simulink model "ball_trajectory"  (R2026a)
settings: Solver=VariableStepAuto  StopTime=5
settings Model: Creator=tdxt  LastModifiedBy=tdxt

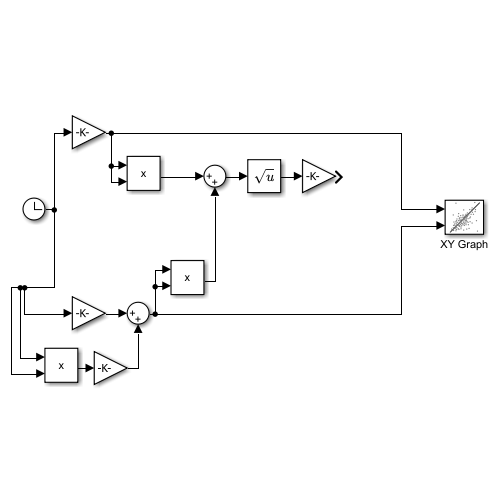
[thumbnail: Simulink's stored preview of the top-level diagram]
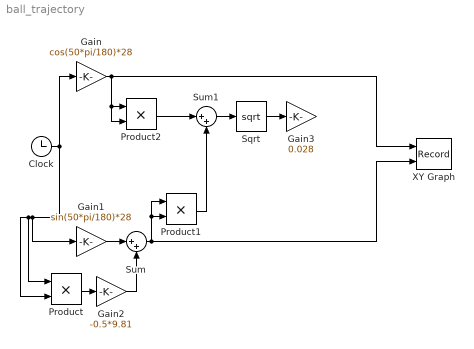
== system ball_trajectory ==
  Clock : Clock
  Gain : Gain  Gain=cos(50*pi/180)*28
  Gain1 : Gain  Gain=sin(50*pi/180)*28
  Gain2 : Gain  Gain=-0.5*9.81
  Gain3 : Gain  Gain=0.028
  Product : Product
  Product1 : Product
  Product2 : Product
  Sqrt : Sqrt
  Sum : Sum  Inputs=|++
  Sum1 : Sum  Inputs=|++
  XY Graph : Record  NumPorts=2.0  FileSettingsInternal="{\"entries\":[{\"content\":{\"excelSettings\":{\"content\":{},\"type\":\"Streamout.ExcelSettings\"},\"parquetSettings\":{\"content\":{},\"type\":\"Streamout.ParquetSettings\"}},\"type\":\"Streamout.FileSettingStorage\",\"uuid\":\"\"}],\"packageUris\":[\"http:\\/\\/schema.mathworks.com\\/mf0\\/streamout_blocks\\/R2020a\"],\"version\":\"1.0\"}"  FrameSettings=[0, 0]  Layout=[1 1]  SignalsInternal="{\"entries\":[{\"content\":{\"signals\":[{\"content\":{\"blockPath\":[],\"dimensions\":[1],\"domain\":\"\",\"lineColor\":\"#a2142f\",\"plots\":[ 1 ],\"port\":1,\"sid\":[\"\"],\"signalID\":1,\"signalName\":\"Gain\"},\"type\":\"RecordBlkView.Signal\",\"uuid\":\"\"},{\"content\":{\"blockPath\":[],\"dimensions\":[1],\"domain\":\"\",\"lineColor\":\"#139fff\",\"plots\":[ 1 ],\"port\":2,\"sid\":[\"\"],\"signalID\":2,\"signalName\":\"Sum\"},\"type\":\"RecordBlkView.Signal\",\"uuid\":\"\"}]},\"type\":\"RecordBlkView.InputSignals\",\"uuid\":\"\"}],\"packageUris\":[\"http:\\/\\/schema.mathworks.com\\/mf0\\/streamout_blocks\\/R2020a\"],\"version\":\"1.0\"}"  VisualizationBindings="{\"xyplotplugin\":{\"info\":[{\"series\":[{\"bindingParametersList\":[{\"parameter\":\"X-Axis\",\"signalID\":1,\"signalName\":\"Gain\"},{\"parameter\":\"Y-Axis\",\"signalID\":2,\"signalName\":\"Sum\"}],\"seriesID\":0}],\"subplotID\":1}]}}"  CompatibilityTag=XY
  wires:
  Clock/1 -> Product/2, Product/1, Gain1/1, Gain/1
  Gain1/1 -> Sum/1
  Gain2/1 -> Sum/2
  Product/1 -> Gain2/1
  Gain/1 -> XY Graph/1, Product2/2, Product2/1
  Sum/1 -> XY Graph/2, Product1/2, Product1/1
  Product2/1 -> Sum1/1
  Product1/1 -> Sum1/2
  Sum1/1 -> Sqrt/1
  Sqrt/1 -> Gain3/1
